simulink library "contactlibV2"  (R2014a)
settings: Solver=ode45  StartTime=0.0  StopTime=10.0  RelTol=1e-3
undefined symbols (not defined in the file): b, b2, k, rWheel, xBlock, yBlock, zBlock
libraries: sm_lib x24, nesl_utility x24, contactlibV2 x10
settings Model: Creator=scastro  LastModifiedBy=scastro

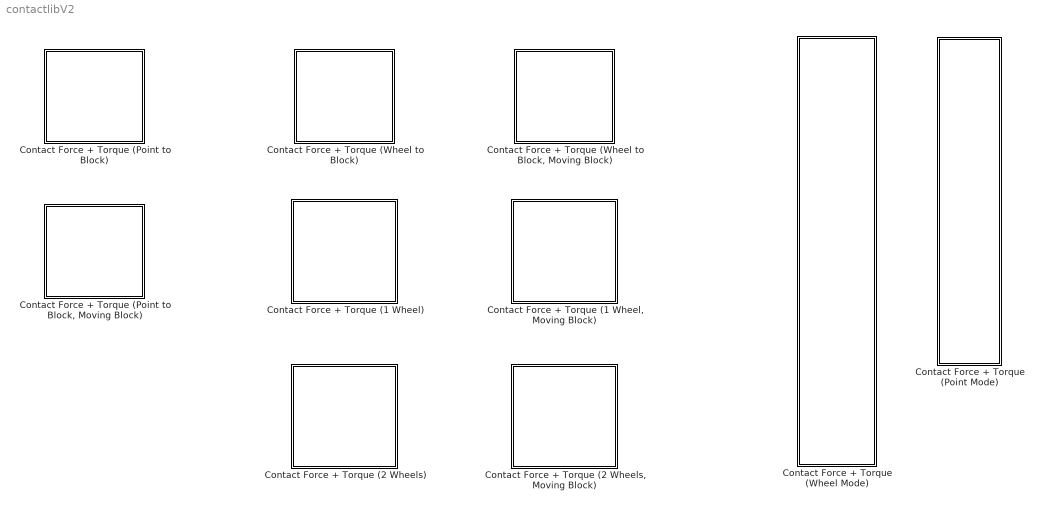
== system contactlibV2 ==
  Contact Force + Torque (1 Wheel) : Subsystem  mask{rWheel=0.1, k=1500, b=25, b2=10, xBlock=30, yBlock=30, zBlock=30, mBlock=5, blockColor=[0.2 0.2 1]}
      mask prompts: rWheel "Wheel Radius [m]"; k "Contact Stiffness [N/m]"; b "Contact Damping [N/(m/s)]"; b2 "Slip Damping [N*s]"; xBlock "Block X [m]"; yBlock "Block Y [m]"; zBlock "Block Z [m]"; mBlock "Block Mass [kg]"; blockColor "Block Color"
  "Contact Force + Torque (1 Wheel, Moving Block)" : Subsystem  mask{rWheel=0.1, k=1500, b=25, b2=10, xBlock=30, yBlock=30, zBlock=30, mBlock=5, blockColor=[0.2 0.2 1]}
      mask prompts: rWheel "Wheel Radius [m]"; k "Contact Stiffness [N/m]"; b "Contact Damping [N/(m/s)]"; b2 "Slip Damping [N*s]"; xBlock "Block X [m]"; yBlock "Block Y [m]"; zBlock "Block Z [m]"; mBlock "Block Mass [kg]"; blockColor "Block Color"
  Contact Force + Torque (2 Wheels) : Subsystem  mask{rWheel=0.1, k=1500, b=25, b2=10, xBlock=30, yBlock=30, zBlock=30, mBlock=5, blockColor=[0.2 0.2 1]}
      mask prompts: rWheel "Wheel Radius [m]"; k "Contact Stiffness [N/m]"; b "Contact Damping [N/(m/s)]"; b2 "Slip Damping [N*s]"; xBlock "Block X [m]"; yBlock "Block Y [m]"; zBlock "Block Z [m]"; mBlock "Block Mass [kg]"; blockColor "Block Color"
  "Contact Force + Torque (2 Wheels, Moving Block)" : Subsystem  mask{rWheel=0.1, k=1500, b=25, b2=10, xBlock=30, yBlock=30, zBlock=30, mBlock=5, blockColor=[0.2 0.2 1]}
      mask prompts: rWheel "Wheel Radius [m]"; k "Contact Stiffness [N/m]"; b "Contact Damping [N/(m/s)]"; b2 "Slip Damping [N*s]"; xBlock "Block X [m]"; yBlock "Block Y [m]"; zBlock "Block Z [m]"; mBlock "Block Mass [kg]"; blockColor "Block Color"
  Contact Force + Torque (Point Mode) : Subsystem
  Contact Force + Torque (Point to Block) : Subsystem  mask{k=1500, b=25, xBlock=20, yBlock=20, zBlock=0.1, mBlock=5, blockColor=[0.2 0.2 1]}
      mask prompts: k "Contact Stiffness [N/m]"; b "Contact Damping [N/(m/s)]"; xBlock "Block X [m]"; yBlock "Block Y [m]"; zBlock "Block Z [m]"; mBlock "Block Mass [kg]"; blockColor "Block Color"
  "Contact Force + Torque (Point to Block, Moving Block)" : Subsystem  mask{k=1500, b=25, xBlock=20, yBlock=20, zBlock=0.1, mBlock=5, blockColor=[0.2 0.2 1]}
      mask prompts: k "Contact Stiffness [N/m]"; b "Contact Damping [N/(m/s)]"; xBlock "Block X [m]"; yBlock "Block Y [m]"; zBlock "Block Z [m]"; mBlock "Block Mass [kg]"; blockColor "Block Color"
  Contact Force + Torque (Wheel Mode) : Subsystem
  Contact Force + Torque (Wheel to Block) : Subsystem  mask{rWheel=0.1, k=1500, b=25, b2=10, xBlock=20, yBlock=20, zBlock=0.1, mBlock=0, blockColor=[0.2 0.2 1]}
      mask prompts: rWheel "Wheel Radius [m]"; k "Contact Stiffness [N/m]"; b "Contact Damping [N/(m/s)]"; b2 "Slip Damping [N*s]"; xBlock "Block X [m]"; yBlock "Block Y [m]"; zBlock "Block Z [m]"; mBlock "Block Mass [kg]"; blockColor "Block Color"
  "Contact Force + Torque (Wheel to Block, Moving Block)" : Subsystem  mask{rWheel=0.1, k=1500, b=25, b2=10, xBlock=20, yBlock=20, zBlock=0.1, mBlock=0, blockColor=[0.2 0.2 1]}
      mask prompts: rWheel "Wheel Radius [m]"; k "Contact Stiffness [N/m]"; b "Contact Damping [N/(m/s)]"; b2 "Slip Damping [N*s]"; xBlock "Block X [m]"; yBlock "Block Y [m]"; zBlock "Block Z [m]"; mBlock "Block Mass [kg]"; blockColor "Block Color"

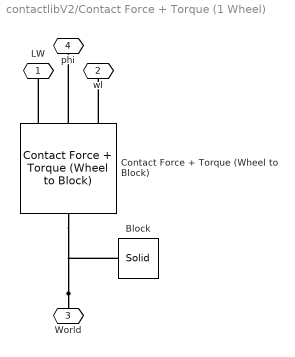
== system contactlibV2/Contact Force + Torque (1 Wheel) ==
  Block : sm_lib/Body Elements/Solid  InertiaType=CalculateFromGeometry  Mass=mBlock  MassUnits=kg  CenterOfMass=[0 0 0]  CenterOfMassUnits=m  MomentsOfInertia=[1 1 1]  MomentsOfInertiaUnits=kg*m^2  ProductsOfInertia=[0 0 0]  ProductsOfInertiaUnits=kg*m^2  DensityBased=off  Density=1000  DensityUnits=kg/(m^3)  GraphicType=FromGeometry  MarkerShape=Sphere  MarkerSize=10  MarkerSizeUnits=m  GraphicVisPropType=SimpleVisualProperties  GraphicDiffuseColor=blockColor  GraphicSpecularColor=[0.5 0.5 0.5 1.0]  GraphicAmbientColor=[0.15 0.15 0.15 1.0]  GraphicEmissiveColor=[0.0 0.0 0.0 1.0]  GraphicShininess=75  GraphicOpacity=1.0  GeometryShape=Brick  RectangleSize=[1 1]  RectangleSizeUnits=m  BrickDimensions=[xBlock yBlock zBlock]  BrickDimensionUnits=m  CylinderRadius=1  CylinderRadiusUnits=m  CylinderLength=1  CylinderLengthUnits=m  SphereRadius=1  SphereRadiusUnits=m  EllipsoidRadii=[1 1 1]  EllipsoidRadiiUnits=m  ExtrusionCrossSection=[1 1; -1 1; -1 -1; 1 -1]  ExtrusionCrossSectionUnits=m  ExtrusionLength=1  ExtrusionLengthUnits=m  PolygonNumSides=3  PolygonOuterRadius=1  PolygonOuterRadiusUnits=m  ExtGeomFileType=STL  ExtGeomFileUnits=m  RevolutionCrossSection=[1 1; 1 -1; 2 -1; 2 1]  RevolutionCrossSectionUnits=m  RevolutionExtent=Full  RevolutionAngle=180  RevolutionAngleUnits=deg  BlockFunction=simmechanics.library.body_elements.solid
  Contact Force + Torque (Wheel to Block) : contactlibV2/Contact Force + Torque (Wheel to Block)  rWheel=rWheel  k=k  b=b  b2=b2  xBlock=xBlock  yBlock=yBlock  zBlock=zBlock  mBlock=mBlock  blockColor=blockColor
  LW : PMIOPort  Port=1  Side=Right
  wl : PMIOPort  Port=2  Side=Right
  World : PMIOPort  Port=3  Side=Left
  phi : PMIOPort  Port=4  Side=Right
  connections:
  Contact Force + Torque (Wheel to Block)/RConn3 -- wl/RConn1
  Contact Force + Torque (Wheel to Block)/RConn1 -- LW/RConn1
  World/RConn1 -- Contact Force + Torque (Wheel to Block)/LConn1 -- Block/RConn1
  Contact Force + Torque (Wheel to Block)/RConn2 -- phi/RConn1

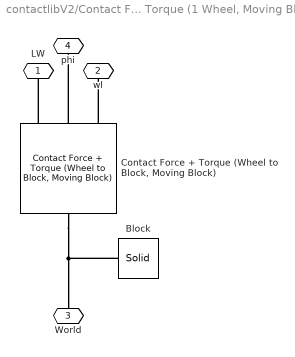
== system contactlibV2/Contact Force + Torque (1 Wheel, Moving Block) ==
  Block : sm_lib/Body Elements/Solid  InertiaType=CalculateFromGeometry  Mass=mBlock  MassUnits=kg  CenterOfMass=[0 0 0]  CenterOfMassUnits=m  MomentsOfInertia=[1 1 1]  MomentsOfInertiaUnits=kg*m^2  ProductsOfInertia=[0 0 0]  ProductsOfInertiaUnits=kg*m^2  DensityBased=off  Density=1000  DensityUnits=kg/(m^3)  GraphicType=FromGeometry  MarkerShape=Sphere  MarkerSize=10  MarkerSizeUnits=m  GraphicVisPropType=SimpleVisualProperties  GraphicDiffuseColor=blockColor  GraphicSpecularColor=[0.5 0.5 0.5 1.0]  GraphicAmbientColor=[0.15 0.15 0.15 1.0]  GraphicEmissiveColor=[0.0 0.0 0.0 1.0]  GraphicShininess=75  GraphicOpacity=1.0  GeometryShape=Brick  RectangleSize=[1 1]  RectangleSizeUnits=m  BrickDimensions=[xBlock yBlock zBlock]  BrickDimensionUnits=m  CylinderRadius=1  CylinderRadiusUnits=m  CylinderLength=1  CylinderLengthUnits=m  SphereRadius=1  SphereRadiusUnits=m  EllipsoidRadii=[1 1 1]  EllipsoidRadiiUnits=m  ExtrusionCrossSection=[1 1; -1 1; -1 -1; 1 -1]  ExtrusionCrossSectionUnits=m  ExtrusionLength=1  ExtrusionLengthUnits=m  PolygonNumSides=3  PolygonOuterRadius=1  PolygonOuterRadiusUnits=m  ExtGeomFileType=STL  ExtGeomFileUnits=m  RevolutionCrossSection=[1 1; 1 -1; 2 -1; 2 1]  RevolutionCrossSectionUnits=m  RevolutionExtent=Full  RevolutionAngle=180  RevolutionAngleUnits=deg  BlockFunction=simmechanics.library.body_elements.solid
  "Contact Force + Torque (Wheel to Block, Moving Block)" : contactlibV2/Contact Force + Torque (Wheel to Block, Moving Block)  rWheel=rWheel  k=k  b=b  b2=b2  xBlock=xBlock  yBlock=yBlock  zBlock=zBlock  mBlock=mBlock  blockColor=blockColor
  LW : PMIOPort  Port=1  Side=Right
  wl : PMIOPort  Port=2  Side=Right
  World : PMIOPort  Port=3  Side=Left
  phi : PMIOPort  Port=4  Side=Right
  connections:
  "Contact Force + Torque (Wheel to Block, Moving Block)"/RConn2 -- phi/RConn1
  Block/RConn1 -- "Contact Force + Torque (Wheel to Block, Moving Block)"/LConn1 -- World/RConn1
  "Contact Force + Torque (Wheel to Block, Moving Block)"/RConn1 -- LW/RConn1
  "Contact Force + Torque (Wheel to Block, Moving Block)"/RConn3 -- wl/RConn1

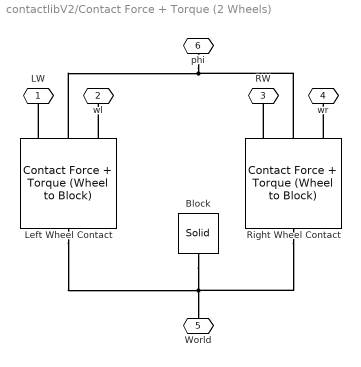
== system contactlibV2/Contact Force + Torque (2 Wheels) ==
  Block : sm_lib/Body Elements/Solid  InertiaType=CalculateFromGeometry  Mass=mBlock  MassUnits=kg  CenterOfMass=[0 0 0]  CenterOfMassUnits=m  MomentsOfInertia=[1 1 1]  MomentsOfInertiaUnits=kg*m^2  ProductsOfInertia=[0 0 0]  ProductsOfInertiaUnits=kg*m^2  DensityBased=off  Density=1000  DensityUnits=kg/(m^3)  GraphicType=FromGeometry  MarkerShape=Sphere  MarkerSize=10  MarkerSizeUnits=m  GraphicVisPropType=SimpleVisualProperties  GraphicDiffuseColor=blockColor  GraphicSpecularColor=[0.5 0.5 0.5 1.0]  GraphicAmbientColor=[0.15 0.15 0.15 1.0]  GraphicEmissiveColor=[0.0 0.0 0.0 1.0]  GraphicShininess=75  GraphicOpacity=1.0  GeometryShape=Brick  RectangleSize=[1 1]  RectangleSizeUnits=m  BrickDimensions=[xBlock yBlock zBlock]  BrickDimensionUnits=m  CylinderRadius=1  CylinderRadiusUnits=m  CylinderLength=1  CylinderLengthUnits=m  SphereRadius=1  SphereRadiusUnits=m  EllipsoidRadii=[1 1 1]  EllipsoidRadiiUnits=m  ExtrusionCrossSection=[1 1; -1 1; -1 -1; 1 -1]  ExtrusionCrossSectionUnits=m  ExtrusionLength=1  ExtrusionLengthUnits=m  PolygonNumSides=3  PolygonOuterRadius=1  PolygonOuterRadiusUnits=m  ExtGeomFileType=STL  ExtGeomFileUnits=m  RevolutionCrossSection=[1 1; 1 -1; 2 -1; 2 1]  RevolutionCrossSectionUnits=m  RevolutionExtent=Full  RevolutionAngle=180  RevolutionAngleUnits=deg  BlockFunction=simmechanics.library.body_elements.solid
  Left Wheel Contact : contactlibV2/Contact Force + Torque (Wheel to Block)  rWheel=rWheel  k=k  b=b  b2=b2  xBlock=xBlock  yBlock=yBlock  zBlock=zBlock  mBlock=mBlock  blockColor=blockColor
  Right Wheel Contact : contactlibV2/Contact Force + Torque (Wheel to Block)  rWheel=rWheel  k=k  b=b  b2=b2  xBlock=xBlock  yBlock=yBlock  zBlock=zBlock  mBlock=mBlock  blockColor=blockColor
  LW : PMIOPort  Port=1  Side=Right
  wl : PMIOPort  Port=2  Side=Right
  RW : PMIOPort  Port=3  Side=Right
  wr : PMIOPort  Port=4  Side=Right
  World : PMIOPort  Port=5  Side=Left
  phi : PMIOPort  Port=6  Side=Right
  connections:
  phi/RConn1 -- Left Wheel Contact/RConn2 -- Right Wheel Contact/RConn2
  Right Wheel Contact/RConn3 -- wr/RConn1
  Block/RConn1 -- Left Wheel Contact/LConn1 -- Right Wheel Contact/LConn1 -- World/RConn1
  Right Wheel Contact/RConn1 -- RW/RConn1
  Left Wheel Contact/RConn1 -- LW/RConn1
  Left Wheel Contact/RConn3 -- wl/RConn1

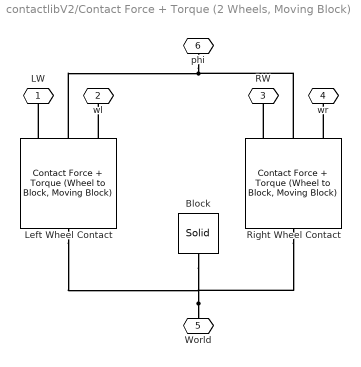
== system contactlibV2/Contact Force + Torque (2 Wheels, Moving Block) ==
  Block : sm_lib/Body Elements/Solid  InertiaType=CalculateFromGeometry  Mass=mBlock  MassUnits=kg  CenterOfMass=[0 0 0]  CenterOfMassUnits=m  MomentsOfInertia=[1 1 1]  MomentsOfInertiaUnits=kg*m^2  ProductsOfInertia=[0 0 0]  ProductsOfInertiaUnits=kg*m^2  DensityBased=off  Density=1000  DensityUnits=kg/(m^3)  GraphicType=FromGeometry  MarkerShape=Sphere  MarkerSize=10  MarkerSizeUnits=m  GraphicVisPropType=SimpleVisualProperties  GraphicDiffuseColor=blockColor  GraphicSpecularColor=[0.5 0.5 0.5 1.0]  GraphicAmbientColor=[0.15 0.15 0.15 1.0]  GraphicEmissiveColor=[0.0 0.0 0.0 1.0]  GraphicShininess=75  GraphicOpacity=1.0  GeometryShape=Brick  RectangleSize=[1 1]  RectangleSizeUnits=m  BrickDimensions=[xBlock yBlock zBlock]  BrickDimensionUnits=m  CylinderRadius=1  CylinderRadiusUnits=m  CylinderLength=1  CylinderLengthUnits=m  SphereRadius=1  SphereRadiusUnits=m  EllipsoidRadii=[1 1 1]  EllipsoidRadiiUnits=m  ExtrusionCrossSection=[1 1; -1 1; -1 -1; 1 -1]  ExtrusionCrossSectionUnits=m  ExtrusionLength=1  ExtrusionLengthUnits=m  PolygonNumSides=3  PolygonOuterRadius=1  PolygonOuterRadiusUnits=m  ExtGeomFileType=STL  ExtGeomFileUnits=m  RevolutionCrossSection=[1 1; 1 -1; 2 -1; 2 1]  RevolutionCrossSectionUnits=m  RevolutionExtent=Full  RevolutionAngle=180  RevolutionAngleUnits=deg  BlockFunction=simmechanics.library.body_elements.solid
  Left Wheel Contact : contactlibV2/Contact Force + Torque (Wheel to Block, Moving Block)  rWheel=rWheel  k=k  b=b  b2=b2  xBlock=xBlock  yBlock=yBlock  zBlock=zBlock  mBlock=mBlock  blockColor=blockColor
  Right Wheel Contact : contactlibV2/Contact Force + Torque (Wheel to Block, Moving Block)  rWheel=rWheel  k=k  b=b  b2=b2  xBlock=xBlock  yBlock=yBlock  zBlock=zBlock  mBlock=mBlock  blockColor=blockColor
  LW : PMIOPort  Port=1  Side=Right
  wl : PMIOPort  Port=2  Side=Right
  RW : PMIOPort  Port=3  Side=Right
  wr : PMIOPort  Port=4  Side=Right
  World : PMIOPort  Port=5  Side=Left
  phi : PMIOPort  Port=6  Side=Right
  connections:
  Left Wheel Contact/RConn3 -- wl/RConn1
  Left Wheel Contact/RConn1 -- LW/RConn1
  Right Wheel Contact/RConn1 -- RW/RConn1
  World/RConn1 -- Left Wheel Contact/LConn1 -- Right Wheel Contact/LConn1 -- Block/RConn1
  Right Wheel Contact/RConn3 -- wr/RConn1
  phi/RConn1 -- Left Wheel Contact/RConn2 -- Right Wheel Contact/RConn2

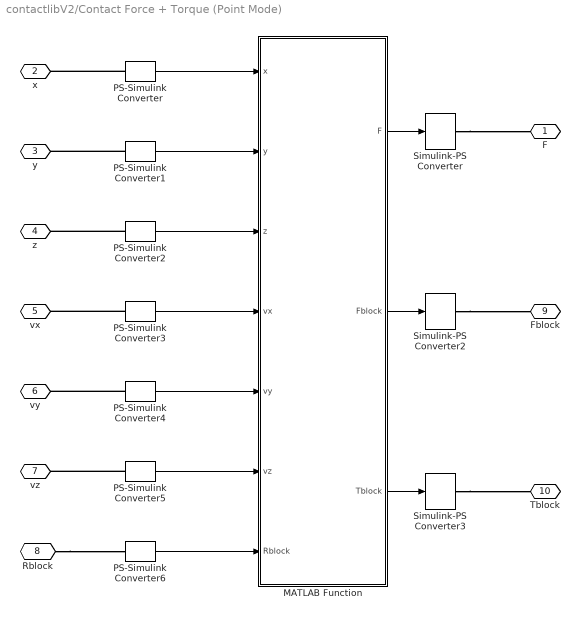
== system contactlibV2/Contact Force + Torque (Point Mode) ==
  MATLAB Function : MATLAB Function  TreatAsAtomicUnit=on
  PS-Simulink Converter{,1..6} (7 alike) : nesl_utility/PS-Simulink Converter  PhysicalDomain=network_engine_domain  SubClassName=ps_output  LeftPortType=input  RightPortType=output  PseudoPeriodic=off  Frequencies=[]  Unit=1  AffineConversion=off
  Simulink-PS Converter : nesl_utility/Simulink-PS Converter  PhysicalDomain=network_engine_domain  SubClassName=ps_input  LeftPortType=input  RightPortType=output  PseudoPeriodic=off  Frequencies=[]  NoiseDistribution=none  NoiseParameters=[]  Unit=1  AffineConversion=off  InputFiltering=off  SimscapeFilterOrder=1  InputFilterTimeConstant=0.001  UdotUserProvided=1
  Simulink-PS Converter2 : nesl_utility/Simulink-PS Converter  PhysicalDomain=network_engine_domain  SubClassName=ps_input  LeftPortType=input  RightPortType=output  PseudoPeriodic=off  Frequencies=[]  NoiseDistribution=none  NoiseParameters=[]  Unit=1  AffineConversion=off  InputFiltering=off  SimscapeFilterOrder=1  InputFilterTimeConstant=0.001  UdotUserProvided=1
  Simulink-PS Converter3 : nesl_utility/Simulink-PS Converter  PhysicalDomain=network_engine_domain  SubClassName=ps_input  LeftPortType=input  RightPortType=output  PseudoPeriodic=off  Frequencies=[]  NoiseDistribution=none  NoiseParameters=[]  Unit=1  AffineConversion=off  InputFiltering=off  SimscapeFilterOrder=1  InputFilterTimeConstant=0.001  UdotUserProvided=1
  F : PMIOPort  Port=1  Side=Right
  x : PMIOPort  Port=2  Side=Left
  y : PMIOPort  Port=3  Side=Left
  z : PMIOPort  Port=4  Side=Left
  vx : PMIOPort  Port=5  Side=Left
  vy : PMIOPort  Port=6  Side=Left
  vz : PMIOPort  Port=7  Side=Left
  Rblock : PMIOPort  Port=8  Side=Left
  Fblock : PMIOPort  Port=9  Side=Right
  Tblock : PMIOPort  Port=10  Side=Right
  wires:
  MATLAB Function/3(Tblock) -> Simulink-PS Converter3/1
  MATLAB Function/2(Fblock) -> Simulink-PS Converter2/1
  PS-Simulink Converter4/1 -> MATLAB Function/5(vy)
  PS-Simulink Converter1/1 -> MATLAB Function/2(y)
  PS-Simulink Converter2/1 -> MATLAB Function/3(z)
  PS-Simulink Converter3/1 -> MATLAB Function/4(vx)
  PS-Simulink Converter5/1 -> MATLAB Function/6(vz)
  PS-Simulink Converter/1 -> MATLAB Function/1(x)
  MATLAB Function/1(F) -> Simulink-PS Converter/1
  PS-Simulink Converter6/1 -> MATLAB Function/7(Rblock)
  connections:
  Simulink-PS Converter3/RConn1 -- Tblock/RConn1
  Simulink-PS Converter2/RConn1 -- Fblock/RConn1
  Simulink-PS Converter/RConn1 -- F/RConn1
  PS-Simulink Converter4/LConn1 -- vy/RConn1
  PS-Simulink Converter/LConn1 -- x/RConn1
  Rblock/RConn1 -- PS-Simulink Converter6/LConn1
  PS-Simulink Converter1/LConn1 -- y/RConn1
  PS-Simulink Converter3/LConn1 -- vx/RConn1
  PS-Simulink Converter2/LConn1 -- z/RConn1
  PS-Simulink Converter5/LConn1 -- vz/RConn1

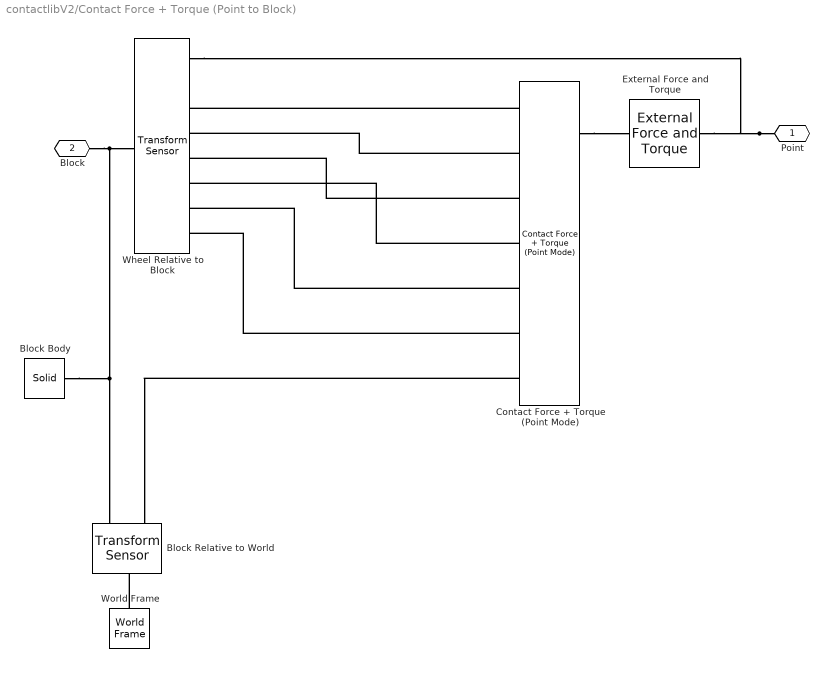
== system contactlibV2/Contact Force + Torque (Point to Block) ==
  Block Body : sm_lib/Body Elements/Solid  InertiaType=CalculateFromGeometry  Mass=mBlock  MassUnits=kg  CenterOfMass=[0 0 0]  CenterOfMassUnits=m  MomentsOfInertia=[1 1 1]  MomentsOfInertiaUnits=kg*m^2  ProductsOfInertia=[0 0 0]  ProductsOfInertiaUnits=kg*m^2  DensityBased=off  Density=1000  DensityUnits=kg/(m^3)  GraphicType=FromGeometry  MarkerShape=Sphere  MarkerSize=10  MarkerSizeUnits=m  GraphicVisPropType=SimpleVisualProperties  GraphicDiffuseColor=blockColor  GraphicSpecularColor=[0.5 0.5 0.5 1.0]  GraphicAmbientColor=[0.15 0.15 0.15 1.0]  GraphicEmissiveColor=[0.0 0.0 0.0 1.0]  GraphicShininess=75  GraphicOpacity=1.0  GeometryShape=Brick  RectangleSize=[1 1]  RectangleSizeUnits=m  BrickDimensions=[xBlock yBlock zBlock]  BrickDimensionUnits=m  CylinderRadius=1  CylinderRadiusUnits=m  CylinderLength=1  CylinderLengthUnits=m  SphereRadius=1  SphereRadiusUnits=m  EllipsoidRadii=[1 1 1]  EllipsoidRadiiUnits=m  ExtrusionCrossSection=[1 1; -1 1; -1 -1; 1 -1]  ExtrusionCrossSectionUnits=m  ExtrusionLength=1  ExtrusionLengthUnits=m  PolygonNumSides=3  PolygonOuterRadius=1  PolygonOuterRadiusUnits=m  ExtGeomFileType=STL  ExtGeomFileUnits=m  RevolutionCrossSection=[1 1; 1 -1; 2 -1; 2 1]  RevolutionCrossSectionUnits=m  RevolutionExtent=Full  RevolutionAngle=180  RevolutionAngleUnits=deg  BlockFunction=simmechanics.library.body_elements.solid
  Block Relative to World : sm_lib/Frames and Transforms/Transform Sensor  MeasurementFrame=Base  SenseAngle=off  SenseAxis=off  SenseAngle1=off  SenseAngle2=off  SenseAngle3=off  SenseQ=off  SenseR=on  SenseOmegaX=off  SenseOmegaY=off  SenseOmegaZ=off  SenseOmega1=off  SenseOmega2=off  SenseOmega3=off  SenseQDot=off  SenseRDot=off  SenseAlphaX=off  SenseAlphaY=off  SenseAlphaZ=off  SenseAlpha1=off  SenseAlpha2=off  SenseAlpha3=off  SenseQDDot=off  SenseRDDot=off  SenseX=off  SenseY=off  SenseZ=off  SenseRad=off  SenseAzim=off  SenseDist=off  SenseInc=off  SenseXDot=off  SenseYDot=off  SenseZDot=off  SenseRadDot=off  SenseAzimDot=off  SenseDistDot=off  SenseIncDot=off  SenseXDDot=off  SenseYDDot=off  SenseZDDot=off  SenseRadDDot=off  SenseAzimDDot=off  SenseDistDDot=off  SenseIncDDot=off  BlockFunction=simmechanics.library.frames_transforms.transform_sensor
  Contact Force + Torque (Point Mode) : contactlibV2/Contact Force + Torque (Point Mode)
  External Force and Torque : sm_lib/Forces and Torques/External Force and Torque  ForceResolutionFrame=World  EnableForceX=off  EnableForceY=off  EnableForceZ=off  EnableForce=on  TorqueResolutionFrame=World  EnableTorqueX=off  EnableTorqueY=off  EnableTorqueZ=off  EnableTorque=off  BlockFunction=simmechanics.library.forces_torques.external_force_torque
  Wheel Relative to Block : sm_lib/Frames and Transforms/Transform Sensor  MeasurementFrame=Base  SenseAngle=off  SenseAxis=off  SenseAngle1=off  SenseAngle2=off  SenseAngle3=off  SenseQ=off  SenseR=on  SenseOmegaX=off  SenseOmegaY=off  SenseOmegaZ=off  SenseOmega1=off  SenseOmega2=off  SenseOmega3=off  SenseQDot=off  SenseRDot=off  SenseAlphaX=off  SenseAlphaY=off  SenseAlphaZ=off  SenseAlpha1=off  SenseAlpha2=off  SenseAlpha3=off  SenseQDDot=off  SenseRDDot=off  SenseX=on  SenseY=on  SenseZ=on  SenseRad=off  SenseAzim=off  SenseDist=off  SenseInc=off  SenseXDot=on  SenseYDot=on  SenseZDot=on  SenseRadDot=off  SenseAzimDot=off  SenseDistDot=off  SenseIncDot=off  SenseXDDot=off  SenseYDDot=off  SenseZDDot=off  SenseRadDDot=off  SenseAzimDDot=off  SenseDistDDot=off  SenseIncDDot=off  BlockFunction=simmechanics.library.frames_transforms.transform_sensor
  World Frame : sm_lib/Frames and Transforms/World Frame  BlockFunction=simmechanics.library.frames_transforms.world_frame
  Point : PMIOPort  Port=1  Side=Right
  Block : PMIOPort  Port=2  Side=Left
  connections:
  World Frame/RConn1 -- Block Relative to World/LConn1
  Point/RConn1 -- External Force and Torque/RConn1 -- Wheel Relative to Block/RConn1
  Block/RConn1 -- Block Relative to World/RConn1 -- Block Body/RConn1 -- Wheel Relative to Block/LConn1
  Contact Force + Torque (Point Mode)/RConn1 -- External Force and Torque/LConn1
  Contact Force + Torque (Point Mode)/LConn1 -- Wheel Relative to Block/RConn3
  Contact Force + Torque (Point Mode)/LConn2 -- Wheel Relative to Block/RConn4
  Contact Force + Torque (Point Mode)/LConn3 -- Wheel Relative to Block/RConn5
  Contact Force + Torque (Point Mode)/LConn4 -- Wheel Relative to Block/RConn6
  Contact Force + Torque (Point Mode)/LConn5 -- Wheel Relative to Block/RConn7
  Contact Force + Torque (Point Mode)/LConn6 -- Wheel Relative to Block/RConn8
  Contact Force + Torque (Point Mode)/LConn7 -- Block Relative to World/RConn2

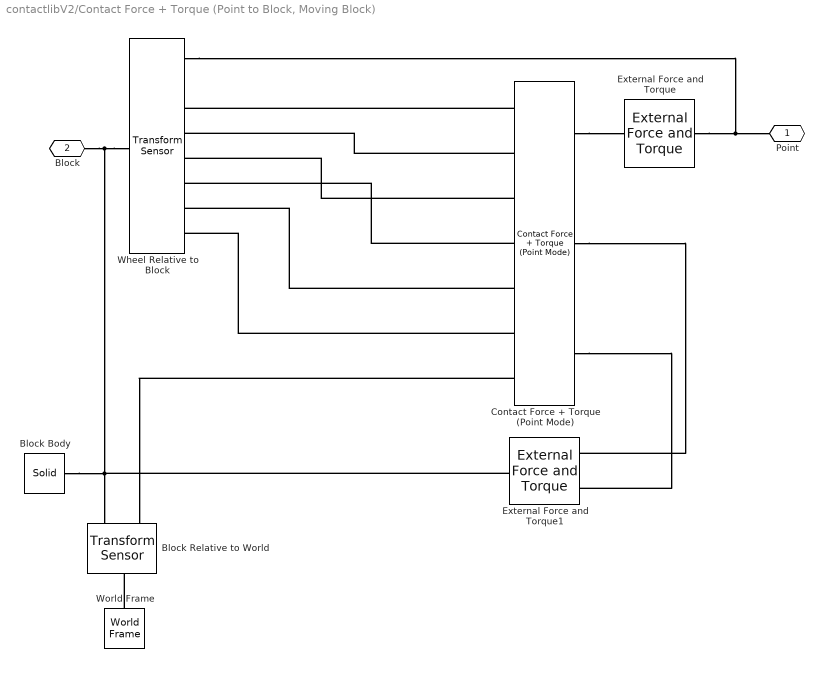
== system contactlibV2/Contact Force + Torque (Point to Block, Moving Block) ==
  Block Body : sm_lib/Body Elements/Solid  InertiaType=CalculateFromGeometry  Mass=mBlock  MassUnits=kg  CenterOfMass=[0 0 0]  CenterOfMassUnits=m  MomentsOfInertia=[1 1 1]  MomentsOfInertiaUnits=kg*m^2  ProductsOfInertia=[0 0 0]  ProductsOfInertiaUnits=kg*m^2  DensityBased=off  Density=1000  DensityUnits=kg/(m^3)  GraphicType=FromGeometry  MarkerShape=Sphere  MarkerSize=10  MarkerSizeUnits=m  GraphicVisPropType=SimpleVisualProperties  GraphicDiffuseColor=blockColor  GraphicSpecularColor=[0.5 0.5 0.5 1.0]  GraphicAmbientColor=[0.15 0.15 0.15 1.0]  GraphicEmissiveColor=[0.0 0.0 0.0 1.0]  GraphicShininess=75  GraphicOpacity=1.0  GeometryShape=Brick  RectangleSize=[1 1]  RectangleSizeUnits=m  BrickDimensions=[xBlock yBlock zBlock]  BrickDimensionUnits=m  CylinderRadius=1  CylinderRadiusUnits=m  CylinderLength=1  CylinderLengthUnits=m  SphereRadius=1  SphereRadiusUnits=m  EllipsoidRadii=[1 1 1]  EllipsoidRadiiUnits=m  ExtrusionCrossSection=[1 1; -1 1; -1 -1; 1 -1]  ExtrusionCrossSectionUnits=m  ExtrusionLength=1  ExtrusionLengthUnits=m  PolygonNumSides=3  PolygonOuterRadius=1  PolygonOuterRadiusUnits=m  ExtGeomFileType=STL  ExtGeomFileUnits=m  RevolutionCrossSection=[1 1; 1 -1; 2 -1; 2 1]  RevolutionCrossSectionUnits=m  RevolutionExtent=Full  RevolutionAngle=180  RevolutionAngleUnits=deg  BlockFunction=simmechanics.library.body_elements.solid
  Block Relative to World : sm_lib/Frames and Transforms/Transform Sensor  MeasurementFrame=Base  SenseAngle=off  SenseAxis=off  SenseAngle1=off  SenseAngle2=off  SenseAngle3=off  SenseQ=off  SenseR=on  SenseOmegaX=off  SenseOmegaY=off  SenseOmegaZ=off  SenseOmega1=off  SenseOmega2=off  SenseOmega3=off  SenseQDot=off  SenseRDot=off  SenseAlphaX=off  SenseAlphaY=off  SenseAlphaZ=off  SenseAlpha1=off  SenseAlpha2=off  SenseAlpha3=off  SenseQDDot=off  SenseRDDot=off  SenseX=off  SenseY=off  SenseZ=off  SenseRad=off  SenseAzim=off  SenseDist=off  SenseInc=off  SenseXDot=off  SenseYDot=off  SenseZDot=off  SenseRadDot=off  SenseAzimDot=off  SenseDistDot=off  SenseIncDot=off  SenseXDDot=off  SenseYDDot=off  SenseZDDot=off  SenseRadDDot=off  SenseAzimDDot=off  SenseDistDDot=off  SenseIncDDot=off  BlockFunction=simmechanics.library.frames_transforms.transform_sensor
  Contact Force + Torque (Point Mode) : contactlibV2/Contact Force + Torque (Point Mode)
  External Force and Torque : sm_lib/Forces and Torques/External Force and Torque  ForceResolutionFrame=World  EnableForceX=off  EnableForceY=off  EnableForceZ=off  EnableForce=on  TorqueResolutionFrame=World  EnableTorqueX=off  EnableTorqueY=off  EnableTorqueZ=off  EnableTorque=off  BlockFunction=simmechanics.library.forces_torques.external_force_torque
  External Force and Torque1 : sm_lib/Forces and Torques/External Force and Torque  ForceResolutionFrame=AttachedFrame  EnableForceX=off  EnableForceY=off  EnableForceZ=off  EnableForce=on  TorqueResolutionFrame=AttachedFrame  EnableTorqueX=off  EnableTorqueY=off  EnableTorqueZ=off  EnableTorque=on  BlockFunction=simmechanics.library.forces_torques.external_force_torque
  Wheel Relative to Block : sm_lib/Frames and Transforms/Transform Sensor  MeasurementFrame=Base  SenseAngle=off  SenseAxis=off  SenseAngle1=off  SenseAngle2=off  SenseAngle3=off  SenseQ=off  SenseR=on  SenseOmegaX=off  SenseOmegaY=off  SenseOmegaZ=off  SenseOmega1=off  SenseOmega2=off  SenseOmega3=off  SenseQDot=off  SenseRDot=off  SenseAlphaX=off  SenseAlphaY=off  SenseAlphaZ=off  SenseAlpha1=off  SenseAlpha2=off  SenseAlpha3=off  SenseQDDot=off  SenseRDDot=off  SenseX=on  SenseY=on  SenseZ=on  SenseRad=off  SenseAzim=off  SenseDist=off  SenseInc=off  SenseXDot=on  SenseYDot=on  SenseZDot=on  SenseRadDot=off  SenseAzimDot=off  SenseDistDot=off  SenseIncDot=off  SenseXDDot=off  SenseYDDot=off  SenseZDDot=off  SenseRadDDot=off  SenseAzimDDot=off  SenseDistDDot=off  SenseIncDDot=off  BlockFunction=simmechanics.library.frames_transforms.transform_sensor
  World Frame : sm_lib/Frames and Transforms/World Frame  BlockFunction=simmechanics.library.frames_transforms.world_frame
  Point : PMIOPort  Port=1  Side=Right
  Block : PMIOPort  Port=2  Side=Left
  connections:
  Contact Force + Torque (Point Mode)/RConn3 -- External Force and Torque1/LConn2
  Contact Force + Torque (Point Mode)/RConn2 -- External Force and Torque1/LConn1
  Contact Force + Torque (Point Mode)/LConn7 -- Block Relative to World/RConn2
  Contact Force + Torque (Point Mode)/LConn6 -- Wheel Relative to Block/RConn8
  Contact Force + Torque (Point Mode)/LConn5 -- Wheel Relative to Block/RConn7
  Contact Force + Torque (Point Mode)/LConn4 -- Wheel Relative to Block/RConn6
  Contact Force + Torque (Point Mode)/LConn3 -- Wheel Relative to Block/RConn5
  Contact Force + Torque (Point Mode)/LConn2 -- Wheel Relative to Block/RConn4
  Contact Force + Torque (Point Mode)/LConn1 -- Wheel Relative to Block/RConn3
  Contact Force + Torque (Point Mode)/RConn1 -- External Force and Torque/LConn1
  Wheel Relative to Block/LConn1 -- External Force and Torque1/RConn1 -- Block Body/RConn1 -- Block Relative to World/RConn1 -- Block/RConn1
  Wheel Relative to Block/RConn1 -- Point/RConn1 -- External Force and Torque/RConn1
  World Frame/RConn1 -- Block Relative to World/LConn1

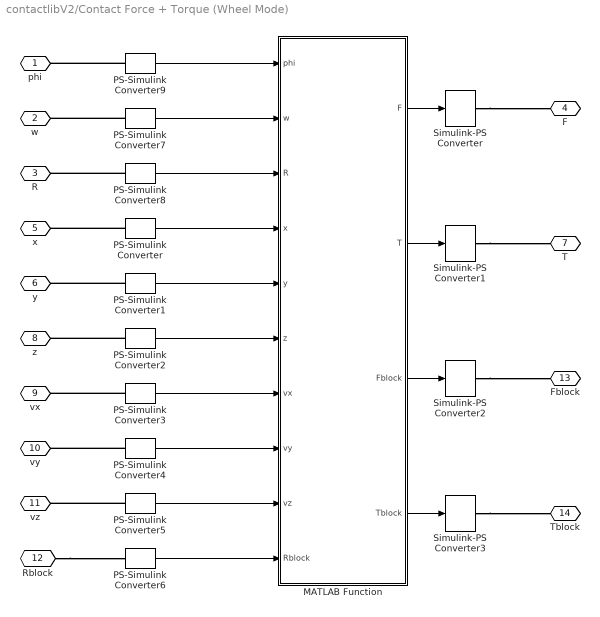
== system contactlibV2/Contact Force + Torque (Wheel Mode) ==
  MATLAB Function : MATLAB Function  TreatAsAtomicUnit=on
  PS-Simulink Converter{,1..9} (10 alike) : nesl_utility/PS-Simulink Converter  PhysicalDomain=network_engine_domain  SubClassName=ps_output  LeftPortType=input  RightPortType=output  PseudoPeriodic=off  Frequencies=[]  Unit=1  AffineConversion=off
  Simulink-PS Converter{,1..3} (4 alike) : nesl_utility/Simulink-PS Converter  PhysicalDomain=network_engine_domain  SubClassName=ps_input  LeftPortType=input  RightPortType=output  PseudoPeriodic=off  Frequencies=[]  NoiseDistribution=none  NoiseParameters=[]  Unit=1  AffineConversion=off  InputFiltering=off  SimscapeFilterOrder=1  InputFilterTimeConstant=0.001  UdotUserProvided=1
  phi : PMIOPort  Port=1  Side=Left
  w : PMIOPort  Port=2  Side=Left
  R : PMIOPort  Port=3  Side=Left
  F : PMIOPort  Port=4  Side=Right
  x : PMIOPort  Port=5  Side=Left
  y : PMIOPort  Port=6  Side=Left
  T : PMIOPort  Port=7  Side=Right
  z : PMIOPort  Port=8  Side=Left
  vx : PMIOPort  Port=9  Side=Left
  vy : PMIOPort  Port=10  Side=Left
  vz : PMIOPort  Port=11  Side=Left
  Rblock : PMIOPort  Port=12  Side=Left
  Fblock : PMIOPort  Port=13  Side=Right
  Tblock : PMIOPort  Port=14  Side=Right
  wires:
  PS-Simulink Converter9/1 -> MATLAB Function/1(phi)
  MATLAB Function/4(Tblock) -> Simulink-PS Converter3/1
  MATLAB Function/3(Fblock) -> Simulink-PS Converter2/1
  PS-Simulink Converter4/1 -> MATLAB Function/8(vy)
  PS-Simulink Converter1/1 -> MATLAB Function/5(y)
  PS-Simulink Converter2/1 -> MATLAB Function/6(z)
  PS-Simulink Converter3/1 -> MATLAB Function/7(vx)
  PS-Simulink Converter8/1 -> MATLAB Function/3(R)
  MATLAB Function/2(T) -> Simulink-PS Converter1/1
  PS-Simulink Converter5/1 -> MATLAB Function/9(vz)
  PS-Simulink Converter/1 -> MATLAB Function/4(x)
  MATLAB Function/1(F) -> Simulink-PS Converter/1
  PS-Simulink Converter7/1 -> MATLAB Function/2(w)
  PS-Simulink Converter6/1 -> MATLAB Function/10(Rblock)
  connections:
  PS-Simulink Converter9/LConn1 -- phi/RConn1
  Simulink-PS Converter3/RConn1 -- Tblock/RConn1
  Simulink-PS Converter2/RConn1 -- Fblock/RConn1
  Simulink-PS Converter/RConn1 -- F/RConn1
  PS-Simulink Converter8/LConn1 -- R/RConn1
  PS-Simulink Converter4/LConn1 -- vy/RConn1
  PS-Simulink Converter7/LConn1 -- w/RConn1
  PS-Simulink Converter/LConn1 -- x/RConn1
  Rblock/RConn1 -- PS-Simulink Converter6/LConn1
  PS-Simulink Converter1/LConn1 -- y/RConn1
  PS-Simulink Converter3/LConn1 -- vx/RConn1
  Simulink-PS Converter1/RConn1 -- T/RConn1
  PS-Simulink Converter2/LConn1 -- z/RConn1
  PS-Simulink Converter5/LConn1 -- vz/RConn1

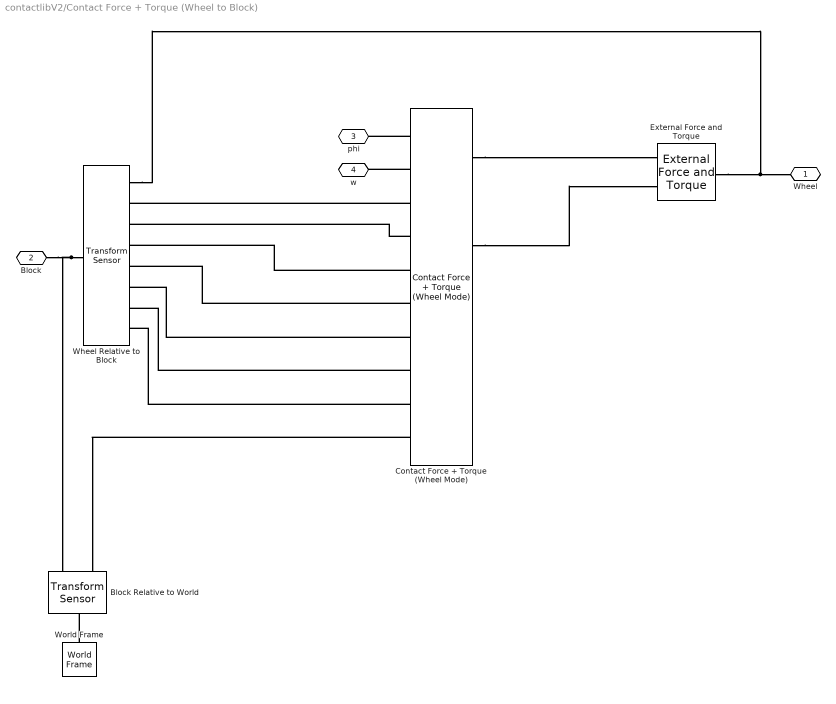
== system contactlibV2/Contact Force + Torque (Wheel to Block) ==
  Block Relative to World : sm_lib/Frames and Transforms/Transform Sensor  MeasurementFrame=Base  SenseAngle=off  SenseAxis=off  SenseAngle1=off  SenseAngle2=off  SenseAngle3=off  SenseQ=off  SenseR=on  SenseOmegaX=off  SenseOmegaY=off  SenseOmegaZ=off  SenseOmega1=off  SenseOmega2=off  SenseOmega3=off  SenseQDot=off  SenseRDot=off  SenseAlphaX=off  SenseAlphaY=off  SenseAlphaZ=off  SenseAlpha1=off  SenseAlpha2=off  SenseAlpha3=off  SenseQDDot=off  SenseRDDot=off  SenseX=off  SenseY=off  SenseZ=off  SenseRad=off  SenseAzim=off  SenseDist=off  SenseInc=off  SenseXDot=off  SenseYDot=off  SenseZDot=off  SenseRadDot=off  SenseAzimDot=off  SenseDistDot=off  SenseIncDot=off  SenseXDDot=off  SenseYDDot=off  SenseZDDot=off  SenseRadDDot=off  SenseAzimDDot=off  SenseDistDDot=off  SenseIncDDot=off  BlockFunction=simmechanics.library.frames_transforms.transform_sensor
  Contact Force + Torque (Wheel Mode) : contactlibV2/Contact Force + Torque (Wheel Mode)
  External Force and Torque : sm_lib/Forces and Torques/External Force and Torque  ForceResolutionFrame=World  EnableForceX=off  EnableForceY=off  EnableForceZ=off  EnableForce=on  TorqueResolutionFrame=World  EnableTorqueX=off  EnableTorqueY=off  EnableTorqueZ=off  EnableTorque=on  BlockFunction=simmechanics.library.forces_torques.external_force_torque
  Wheel Relative to Block : sm_lib/Frames and Transforms/Transform Sensor  MeasurementFrame=Base  SenseAngle=off  SenseAxis=off  SenseAngle1=off  SenseAngle2=off  SenseAngle3=off  SenseQ=off  SenseR=on  SenseOmegaX=off  SenseOmegaY=off  SenseOmegaZ=off  SenseOmega1=off  SenseOmega2=off  SenseOmega3=off  SenseQDot=off  SenseRDot=off  SenseAlphaX=off  SenseAlphaY=off  SenseAlphaZ=off  SenseAlpha1=off  SenseAlpha2=off  SenseAlpha3=off  SenseQDDot=off  SenseRDDot=off  SenseX=on  SenseY=on  SenseZ=on  SenseRad=off  SenseAzim=off  SenseDist=off  SenseInc=off  SenseXDot=on  SenseYDot=on  SenseZDot=on  SenseRadDot=off  SenseAzimDot=off  SenseDistDot=off  SenseIncDot=off  SenseXDDot=off  SenseYDDot=off  SenseZDDot=off  SenseRadDDot=off  SenseAzimDDot=off  SenseDistDDot=off  SenseIncDDot=off  BlockFunction=simmechanics.library.frames_transforms.transform_sensor
  World Frame : sm_lib/Frames and Transforms/World Frame  BlockFunction=simmechanics.library.frames_transforms.world_frame
  Wheel : PMIOPort  Port=1  Side=Right
  Block : PMIOPort  Port=2  Side=Left
  phi : PMIOPort  Port=3  Side=Right
  w : PMIOPort  Port=4  Side=Right
  connections:
  Contact Force + Torque (Wheel Mode)/LConn10 -- Block Relative to World/RConn2
  Contact Force + Torque (Wheel Mode)/LConn9 -- Wheel Relative to Block/RConn8
  Contact Force + Torque (Wheel Mode)/LConn8 -- Wheel Relative to Block/RConn7
  Contact Force + Torque (Wheel Mode)/LConn7 -- Wheel Relative to Block/RConn6
  Contact Force + Torque (Wheel Mode)/LConn6 -- Wheel Relative to Block/RConn5
  Contact Force + Torque (Wheel Mode)/LConn5 -- Wheel Relative to Block/RConn4
  Contact Force + Torque (Wheel Mode)/LConn4 -- Wheel Relative to Block/RConn3
  Contact Force + Torque (Wheel Mode)/LConn3 -- Wheel Relative to Block/RConn2
  Contact Force + Torque (Wheel Mode)/LConn1 -- phi/RConn1
  Contact Force + Torque (Wheel Mode)/LConn2 -- w/RConn1
  Contact Force + Torque (Wheel Mode)/RConn2 -- External Force and Torque/LConn2
  Contact Force + Torque (Wheel Mode)/RConn1 -- External Force and Torque/LConn1
  Wheel Relative to Block/LConn1 -- Block Relative to World/RConn1 -- Block/RConn1
  Wheel Relative to Block/RConn1 -- Wheel/RConn1 -- External Force and Torque/RConn1
  World Frame/RConn1 -- Block Relative to World/LConn1

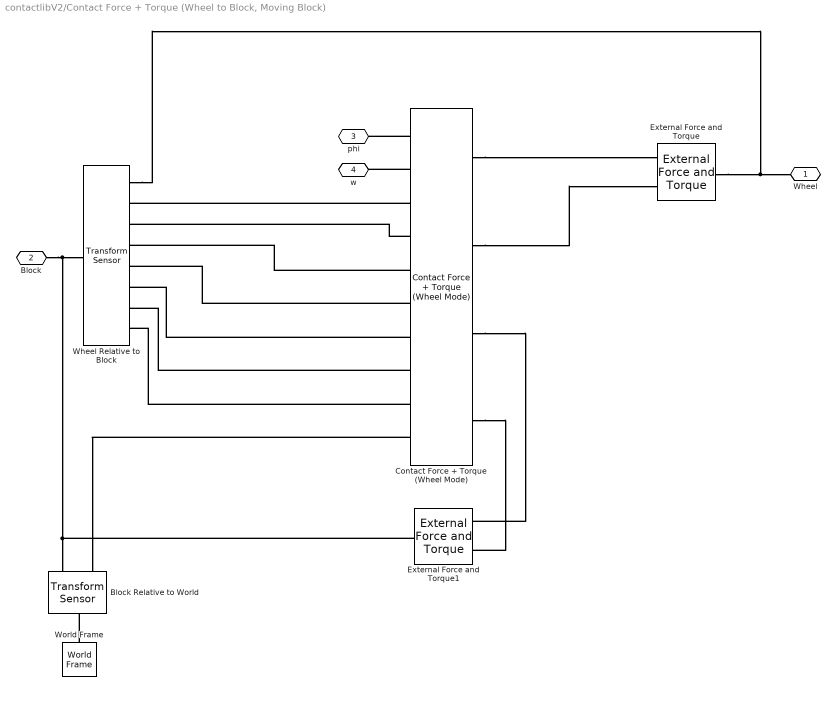
== system contactlibV2/Contact Force + Torque (Wheel to Block, Moving Block) ==
  Block Relative to World : sm_lib/Frames and Transforms/Transform Sensor  MeasurementFrame=Base  SenseAngle=off  SenseAxis=off  SenseAngle1=off  SenseAngle2=off  SenseAngle3=off  SenseQ=off  SenseR=on  SenseOmegaX=off  SenseOmegaY=off  SenseOmegaZ=off  SenseOmega1=off  SenseOmega2=off  SenseOmega3=off  SenseQDot=off  SenseRDot=off  SenseAlphaX=off  SenseAlphaY=off  SenseAlphaZ=off  SenseAlpha1=off  SenseAlpha2=off  SenseAlpha3=off  SenseQDDot=off  SenseRDDot=off  SenseX=off  SenseY=off  SenseZ=off  SenseRad=off  SenseAzim=off  SenseDist=off  SenseInc=off  SenseXDot=off  SenseYDot=off  SenseZDot=off  SenseRadDot=off  SenseAzimDot=off  SenseDistDot=off  SenseIncDot=off  SenseXDDot=off  SenseYDDot=off  SenseZDDot=off  SenseRadDDot=off  SenseAzimDDot=off  SenseDistDDot=off  SenseIncDDot=off  BlockFunction=simmechanics.library.frames_transforms.transform_sensor
  Contact Force + Torque (Wheel Mode) : contactlibV2/Contact Force + Torque (Wheel Mode)
  External Force and Torque : sm_lib/Forces and Torques/External Force and Torque  ForceResolutionFrame=World  EnableForceX=off  EnableForceY=off  EnableForceZ=off  EnableForce=on  TorqueResolutionFrame=World  EnableTorqueX=off  EnableTorqueY=off  EnableTorqueZ=off  EnableTorque=on  BlockFunction=simmechanics.library.forces_torques.external_force_torque
  External Force and Torque1 : sm_lib/Forces and Torques/External Force and Torque  ForceResolutionFrame=AttachedFrame  EnableForceX=off  EnableForceY=off  EnableForceZ=off  EnableForce=on  TorqueResolutionFrame=AttachedFrame  EnableTorqueX=off  EnableTorqueY=off  EnableTorqueZ=off  EnableTorque=on  BlockFunction=simmechanics.library.forces_torques.external_force_torque
  Wheel Relative to Block : sm_lib/Frames and Transforms/Transform Sensor  MeasurementFrame=Base  SenseAngle=off  SenseAxis=off  SenseAngle1=off  SenseAngle2=off  SenseAngle3=off  SenseQ=off  SenseR=on  SenseOmegaX=off  SenseOmegaY=off  SenseOmegaZ=off  SenseOmega1=off  SenseOmega2=off  SenseOmega3=off  SenseQDot=off  SenseRDot=off  SenseAlphaX=off  SenseAlphaY=off  SenseAlphaZ=off  SenseAlpha1=off  SenseAlpha2=off  SenseAlpha3=off  SenseQDDot=off  SenseRDDot=off  SenseX=on  SenseY=on  SenseZ=on  SenseRad=off  SenseAzim=off  SenseDist=off  SenseInc=off  SenseXDot=on  SenseYDot=on  SenseZDot=on  SenseRadDot=off  SenseAzimDot=off  SenseDistDot=off  SenseIncDot=off  SenseXDDot=off  SenseYDDot=off  SenseZDDot=off  SenseRadDDot=off  SenseAzimDDot=off  SenseDistDDot=off  SenseIncDDot=off  BlockFunction=simmechanics.library.frames_transforms.transform_sensor
  World Frame : sm_lib/Frames and Transforms/World Frame  BlockFunction=simmechanics.library.frames_transforms.world_frame
  Wheel : PMIOPort  Port=1  Side=Right
  Block : PMIOPort  Port=2  Side=Left
  phi : PMIOPort  Port=3  Side=Right
  w : PMIOPort  Port=4  Side=Right
  connections:
  World Frame/RConn1 -- Block Relative to World/LConn1
  External Force and Torque/RConn1 -- Wheel/RConn1 -- Wheel Relative to Block/RConn1
  Block/RConn1 -- External Force and Torque1/RConn1 -- Block Relative to World/RConn1 -- Wheel Relative to Block/LConn1
  Contact Force + Torque (Wheel Mode)/RConn1 -- External Force and Torque/LConn1
  Contact Force + Torque (Wheel Mode)/RConn2 -- External Force and Torque/LConn2
  Contact Force + Torque (Wheel Mode)/LConn2 -- w/RConn1
  Contact Force + Torque (Wheel Mode)/LConn1 -- phi/RConn1
  Contact Force + Torque (Wheel Mode)/LConn3 -- Wheel Relative to Block/RConn2
  Contact Force + Torque (Wheel Mode)/LConn4 -- Wheel Relative to Block/RConn3
  Contact Force + Torque (Wheel Mode)/LConn5 -- Wheel Relative to Block/RConn4
  Contact Force + Torque (Wheel Mode)/LConn6 -- Wheel Relative to Block/RConn5
  Contact Force + Torque (Wheel Mode)/LConn7 -- Wheel Relative to Block/RConn6
  Contact Force + Torque (Wheel Mode)/LConn8 -- Wheel Relative to Block/RConn7
  Contact Force + Torque (Wheel Mode)/LConn9 -- Wheel Relative to Block/RConn8
  Contact Force + Torque (Wheel Mode)/LConn10 -- Block Relative to World/RConn2
  Contact Force + Torque (Wheel Mode)/RConn3 -- External Force and Torque1/LConn1
  Contact Force + Torque (Wheel Mode)/RConn4 -- External Force and Torque1/LConn2

== matlab function contactlibV2/Contact Force + Torque (Point Mode)/MATLAB Function ==
  data: x input; y input; z input; vx input; vy input; vz input; Rblock input; zBlock parameter; F output size=3; k parameter; b parameter; yBlock parameter; xBlock parameter; b2 parameter; Fblock output; Tblock output
function [F,Fblock,Tblock] = contact(x,y,z,vx,vy,vz,Rblock, zBlock, k, b, yBlock, xBlock, b2)
%#codegen

%% FUNCTION INTERFACE DESCRIPTION

% OUTPUTS:
% F:  Force applied to point, in world coordinates
% Fblock:  Force applied to block, in block coordinates
% Tblock:  Torque applied to block, in block coordinates

% INPUTS:
% x,y,z:  Translational position of point relative to Block
% vx,vy,vz:  Translational velocity of point relative to Block
% Rblock:  Rotation matrix of Block relative to World

% PARAMETERS:
% xBlock, yBlock, zBlock:  Block dimensions
% k:  Contact stiffness
% b:  Contact damping
% b2:  Friction damping

%% Initialize 3-D quantities
F = zeros(3,1);

%% Big if-statement
% UPPER (Z) SURFACE
if  z < zBlock/2 && ...
   (x>-xBlock/2) && (x<xBlock/2) && ...
   (y>-yBlock/2) && (y<yBlock/2) && (z>0)

    % Normal contact force: Acts upwards along z-direction
    F(3) = k*( zBlock/2 - z ) -b*vz;
end

%% Rotate forces back to world coordinates
F = Rblock*F;
Fblock = -F;
Tblock = [0 -z y ; z 0 -x; -y x 0]*Fblock;

== matlab function contactlibV2/Contact Force + Torque (Wheel Mode)/MATLAB Function ==
  data: phi input; w input; R input; x input; y input; z input; vx input; vy input; vz input; Rblock input; zBlock parameter; rWheel parameter; F output size=3; k parameter; b parameter; yBlock parameter; xBlock parameter; b2 parameter; T output; Fblock output; Tblock output
function [F,T,Fblock,Tblock] = contact_force_torque(phi,w,R,x,y,z,vx,vy,vz,Rblock, zBlock, rWheel, k, b, yBlock, xBlock, b2)
%#codegen

%% FUNCTION INTERFACE DESCRIPTION

% OUTPUTS:
% F:  Force applied to wheel, in world coordinates
% T:  Torque applied to wheel, in world coordinates
% Fblock:  Force applied to block, in block coordinates
% Tblock:  Torque applied to block, in block coordinates

% INPUTS:
% phi:  Angle that the robot makes with the world x-axis
% w:  Wheel angular velocity
% R:  Rotation matrix of Wheel relative to Block
% x,y,z:  Translational position of Wheel relative to Block
% vx,vy,vz:  Translational velocity of Wheel relative to Block
% Rblock:  Rotation matrix of Block relative to World

% PARAMETERS:
% xBlock, yBlock, zBlock:  Block dimensions
% rWheel:  Wheel radius
% k:  Contact stiffness
% b:  Contact damping
% b2:  Friction damping

%% Initialize 3-D quantities
F = zeros(3,1);
T = zeros(3,1);
wVec = R*[0;0;w];

%% Big if-statement
% UPPER (Z) SURFACE
if (z - rWheel) < zBlock/2 && ...
   (x>-xBlock/2) && (x<xBlock/2) && ...
   (y>-yBlock/2) && (y<yBlock/2) && (z>0)

    % Normal contact force: Acts upwards along z-direction
    F(3) = k*( zBlock/2 - z + rWheel ) -b*vz;

    % Friction torque: Should cause the wheel to spin in the same place it moves.
    T(1) = b2*(-vy - wVec(1)*rWheel);
    T(2) = b2*(vx - wVec(2)*rWheel);   
  
    % Friction forces:  Since force is applied at the contact point
    F(1) = F(1) - T(2)/rWheel;
    F(2) = F(2) + T(1)/rWheel;

% UPPER RIGHT (XZ) CORNER
elseif (y>-yBlock/2) && (y<yBlock/2) && ...
       (x>xBlock/2)  && (z>zBlock/2) && ...
       ((x-xBlock/2)^2 + (z-zBlock/2)^2 < (rWheel*cos(phi))^2)
    
    theta = atan2(z-zBlock/2,x-xBlock/2);

    % Normal contact force: 
    % Acts upwards along z-direction and right along x-direction.
    F(3) = k*( zBlock/2 - z + rWheel*sin(theta) ) -b*vz;
    Flat = F(3)/tan(theta);
    F(1) = Flat*abs(cos(phi));
    F(2) = -Flat*sin(phi);
    
    % Friction torque: Should cause the wheel to spin in the same place it moves.
    T(1) = b2*(-vy - wVec(1)*rWheel);
    T(2) = b2*(vx - wVec(2)*rWheel);   
  
    % Friction forces:  Since force is applied at the contact point
    F(1) = F(1) - T(2)/(rWheel*sin(theta));
    F(2) = F(2) + T(1)/(rWheel*sin(theta));
    
% UPPER LEFT (XZ) CORNER
elseif (y>-yBlock/2) && (y<yBlock/2) && ...
       (x<-xBlock/2)  && (z>zBlock/2) && ...
       ((-xBlock/2-x)^2 + (z-zBlock/2)^2 < (rWheel*cos(phi))^2)
    
    theta = atan2(z-zBlock/2,-xBlock/2-x);

    % Normal contact force: 
    % Acts upwards along z-direction and right along x-direction.
    F(3) = k*( zBlock/2 - z + rWheel*sin(theta) ) -b*vz;
    Flat = -F(3)/tan(theta);
    F(1) = Flat*abs(cos(phi));
    F(2) = -Flat*sin(phi);
    
    % Friction torque: Should cause the wheel to spin in the same place it moves.
    T(1) = b2*(-vy - wVec(1)*rWheel);
    T(2) = b2*(vx - wVec(2)*rWheel);   
  
    % Friction forces:  Since force is applied at the contact point
    F(1) = F(1) - T(2)/(rWheel*sin(theta));
    F(2) = F(2) + T(1)/(rWheel*sin(theta));
   
end

%% Rotate forces back to world coordinates
F = Rblock*F;
T = Rblock*T;
Fblock = -F;
Tblock = [0 -z y ; z 0 -x; -y x 0]*Fblock;
